simulink model "taetEMIL"  (R2021a)
settings: Solver=VariableStepAuto  StartTime=0.0  StopTime=2* 60*60  RelTol=1e-3
values from neighbouring files (symbols this model uses):
  Battery_Capacity = 100000    [load_global_variables.m]
  SOC_Start = 50    [load_global_variables.m]
  T_bat = 30*60    (= 1800)    [load_global_variables.m]
libraries: simulink x1
settings Model: Creator=cm  LastModifiedBy=cm

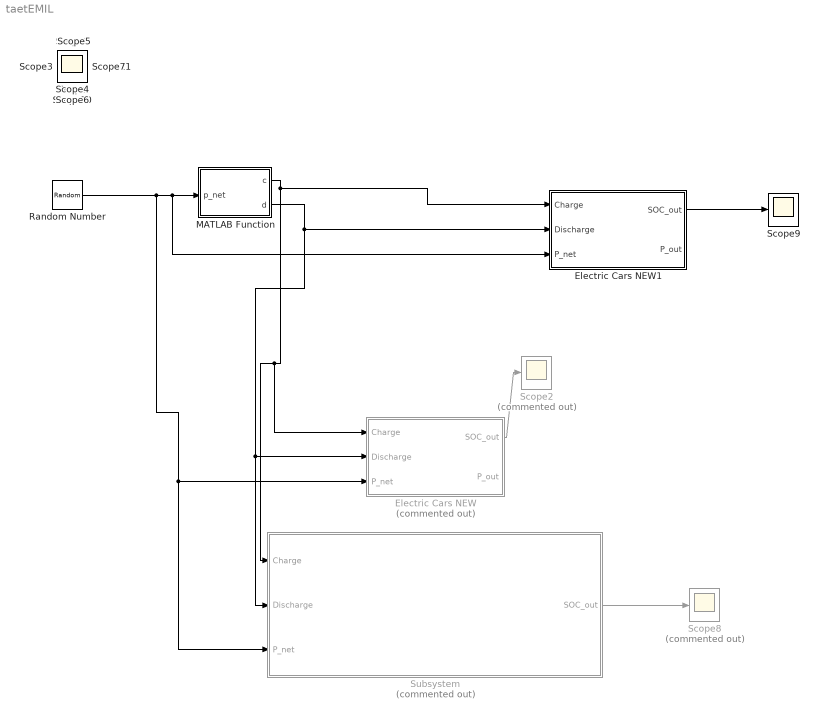
== system taetEMIL ==
  Electric Cars NEW : Subsystem  Commented=on
  Electric Cars NEW1 : Subsystem
  MATLAB Function : MATLAB Function  TreatAsAtomicUnit=on
  Random Number : RandomNumber  Variance=1000  SampleTime=10*60
  Scope2 : Scope  Commented=on
  Scope8 : Scope  Commented=on
  Scope{,1,3..7,9..11} (10 alike) : Scope
  Subsystem : Subsystem  Commented=on
  wires:
  MATLAB Function/1(c) -> Electric Cars NEW1/1(Charge), Subsystem/1(Charge), Electric Cars NEW/1(Charge)
  MATLAB Function/2(d) -> Electric Cars NEW1/2(Discharge), Subsystem/2(Discharge), Electric Cars NEW/2(Discharge)
  Electric Cars NEW/1(SOC_out) -> Scope2/1
  Random Number/1 -> Subsystem/3(P_net), Electric Cars NEW/3(P_net), Electric Cars NEW1/3(P_net), MATLAB Function/1(p_net)
  Subsystem/1(SOC_out) -> Scope8/1
  Electric Cars NEW1/1(SOC_out) -> Scope9/1

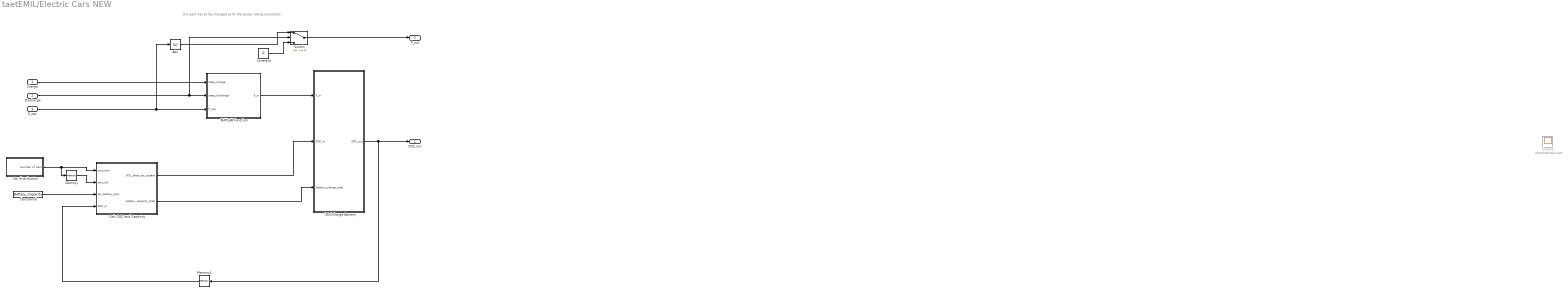
== system taetEMIL/Electric Cars NEW ==
  note: this part has to be changed to fit the power rating constraint
  Charge : Inport
  Discharge : Inport  Port=2
  P_net : Inport  Port=3
  (Dis)Charge Battery : Subsystem
  Abs : Abs
  Calc SOC and Capacity : MATLAB Function  TreatAsAtomicUnit=on
  Car distribution : Subsystem  TreatAsAtomicUnit=on
  Constant : Constant  Value=0
  Constant6 : Constant  Value=Battery_Capacity
  MATLAB Function : MATLAB Function  TreatAsAtomicUnit=on
  Memory : Memory  InitialCondition=100
  Memory1 : Memory  InitialCondition=SOC_Start
  Scope9 : Scope  Commented=on
  Switch : Switch  Criteria=u2 ~= 0
  SOC_out : Outport
  P_out : Outport  Port=2
  wires:
  Car distribution/1(Number of Cars) -> Memory/1, Calc SOC and Capacity/1(cars_new)
  Memory/1 -> Calc SOC and Capacity/2(cars_old)
  Constant6/1 -> Calc SOC and Capacity/3(car_battery_size)
  Memory1/1 -> Calc SOC and Capacity/4(SOC_in)
  MATLAB Function/1(P_in) -> (Dis)Charge Battery/1(P_in)
  Calc SOC and Capacity/1(SOC_after_car_update) -> (Dis)Charge Battery/2(SOC_in)
  Calc SOC and Capacity/2(battery_capacity_total) -> (Dis)Charge Battery/3(battery_charge_total)
  P_net/1 -> Abs/1, MATLAB Function/3(P_net)
  Discharge/1 -> Switch/2, MATLAB Function/2(state_discharge)
  Charge/1 -> MATLAB Function/1(state_charge)
  (Dis)Charge Battery/1(SOC_out) -> Memory1/1, SOC_out/1
  Abs/1 -> Switch/1
  Constant/1 -> Switch/3
  Switch/1 -> P_out/1

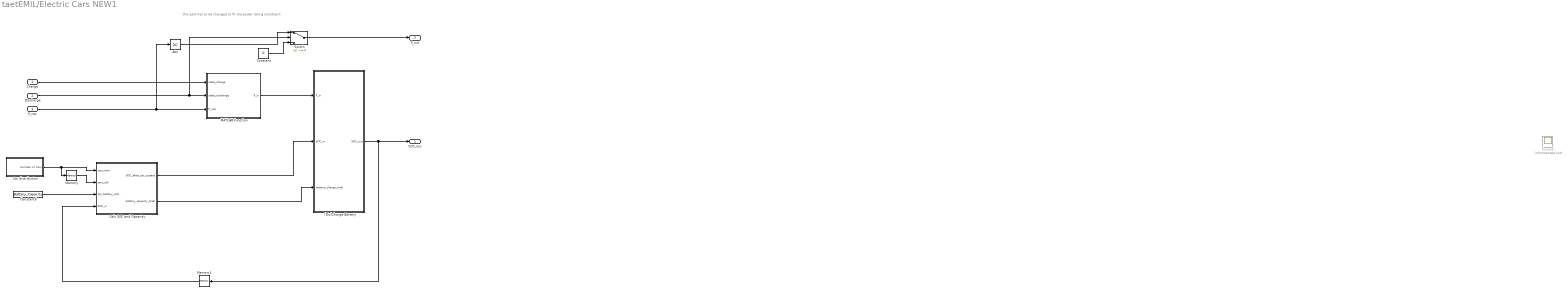
== system taetEMIL/Electric Cars NEW1 ==
  note: this part has to be changed to fit the power rating constraint
  Charge : Inport
  Discharge : Inport  Port=2
  P_net : Inport  Port=3
  (Dis)Charge Battery : Subsystem
  Abs : Abs
  Calc SOC and Capacity : MATLAB Function  TreatAsAtomicUnit=on
  Car distribution : Subsystem  TreatAsAtomicUnit=on
  Constant : Constant  Value=0
  Constant6 : Constant  Value=Battery_Capacity
  MATLAB Function : MATLAB Function  TreatAsAtomicUnit=on
  Memory : Memory  InitialCondition=1
  Memory1 : Memory  InitialCondition=SOC_Start
  Scope9 : Scope  Commented=on
  Switch : Switch  Criteria=u2 ~= 0
  SOC_out : Outport
  P_out : Outport  Port=2
  wires:
  Car distribution/1(Number of Cars) -> Memory/1, Calc SOC and Capacity/1(cars_new)
  Memory/1 -> Calc SOC and Capacity/2(cars_old)
  Constant6/1 -> Calc SOC and Capacity/3(car_battery_size)
  Memory1/1 -> Calc SOC and Capacity/4(SOC_in)
  MATLAB Function/1(P_in) -> (Dis)Charge Battery/1(P_in)
  Calc SOC and Capacity/1(SOC_after_car_update) -> (Dis)Charge Battery/2(SOC_in)
  Calc SOC and Capacity/2(battery_capacity_total) -> (Dis)Charge Battery/3(battery_charge_total)
  P_net/1 -> Abs/1, MATLAB Function/3(P_net)
  Discharge/1 -> Switch/2, MATLAB Function/2(state_discharge)
  Charge/1 -> MATLAB Function/1(state_charge)
  (Dis)Charge Battery/1(SOC_out) -> Memory1/1, SOC_out/1
  Abs/1 -> Switch/1
  Constant/1 -> Switch/3
  Switch/1 -> P_out/1

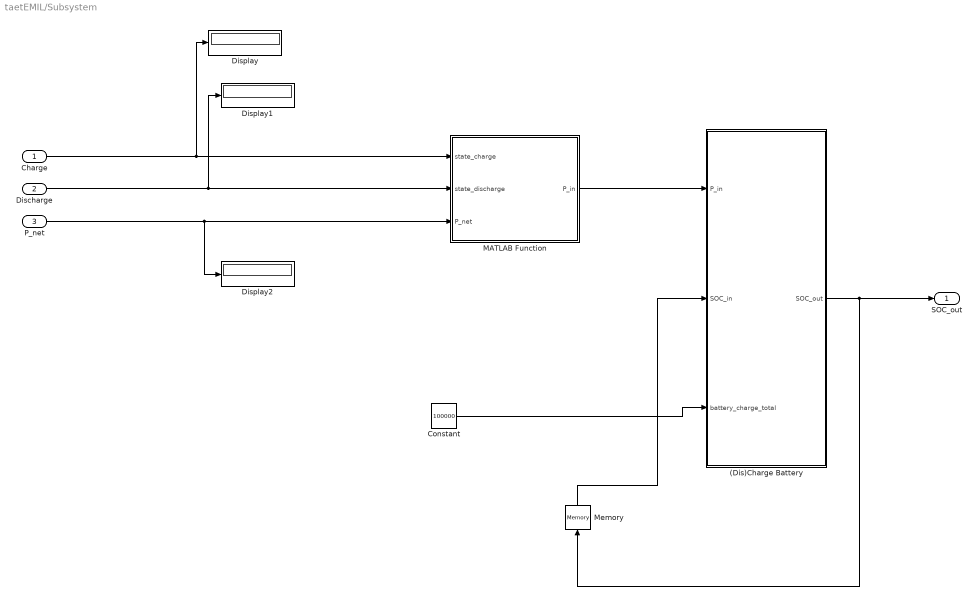
== system taetEMIL/Subsystem ==
  Charge : Inport
  Discharge : Inport  Port=2
  P_net : Inport  Port=3
  (Dis)Charge Battery : Subsystem
  Constant : Constant  Value=100000
  Display : Display
  Display1 : Display
  Display2 : Display
  MATLAB Function : MATLAB Function  TreatAsAtomicUnit=on
  Memory : Memory  InitialCondition=50
  SOC_out : Outport
  wires:
  Charge/1 -> Display/1, MATLAB Function/1(state_charge)
  MATLAB Function/1(P_in) -> (Dis)Charge Battery/1(P_in)
  P_net/1 -> Display2/1, MATLAB Function/3(P_net)
  Discharge/1 -> Display1/1, MATLAB Function/2(state_discharge)
  Memory/1 -> (Dis)Charge Battery/2(SOC_in)
  (Dis)Charge Battery/1(SOC_out) -> Memory/1, SOC_out/1
  Constant/1 -> (Dis)Charge Battery/3(battery_charge_total)

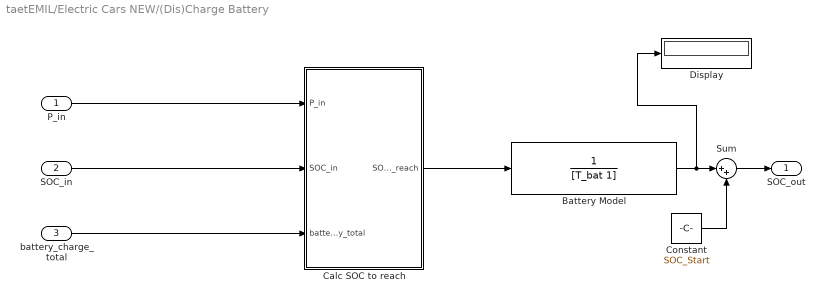
== system taetEMIL/Electric Cars NEW/(Dis)Charge Battery ==
  P_in : Inport
  SOC_in : Inport  Port=2
  battery_charge_total : Inport  Port=3
  Battery Model : TransferFcn  Numerator=1  Denominator=[T_bat 1]
  Calc SOC to reach : MATLAB Function  TreatAsAtomicUnit=on
  Constant : Constant  Value=SOC_Start
  Display : Display
  Sum : Sum  Inputs=|++
  SOC_out : Outport
  wires:
  Calc SOC to reach/1(SOC_to_reach) -> Battery Model/1
  P_in/1 -> Calc SOC to reach/1(P_in)
  SOC_in/1 -> Calc SOC to reach/2(SOC_in)
  battery_charge_total/1 -> Calc SOC to reach/3(battery_capacity_total)
  Sum/1 -> SOC_out/1
  Battery Model/1 -> Display/1, Sum/1
  Constant/1 -> Sum/2

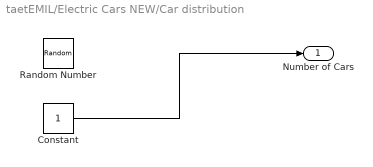
== system taetEMIL/Electric Cars NEW/Car distribution ==
  Constant : Constant
  Random Number : RandomNumber  Mean=50  Variance=15  SampleTime=10*60
  Number of Cars : Outport
  wires:
  Constant/1 -> Number of Cars/1

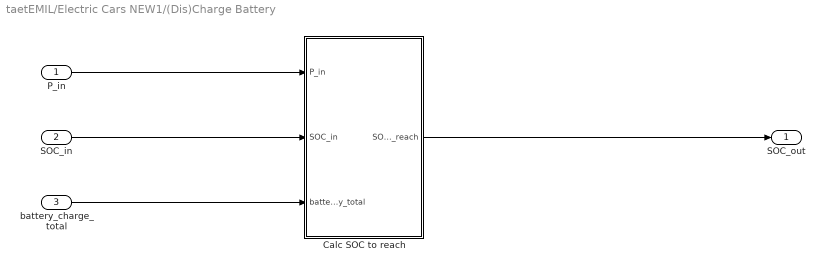
== system taetEMIL/Electric Cars NEW1/(Dis)Charge Battery ==
  P_in : Inport
  SOC_in : Inport  Port=2
  battery_charge_total : Inport  Port=3
  Calc SOC to reach : MATLAB Function  TreatAsAtomicUnit=on
  SOC_out : Outport
  wires:
  P_in/1 -> Calc SOC to reach/1(P_in)
  SOC_in/1 -> Calc SOC to reach/2(SOC_in)
  battery_charge_total/1 -> Calc SOC to reach/3(battery_capacity_total)
  Calc SOC to reach/1(SOC_to_reach) -> SOC_out/1

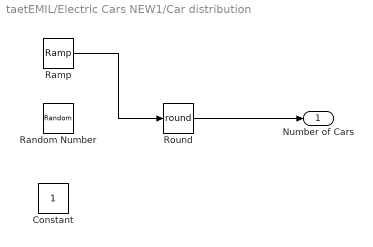
== system taetEMIL/Electric Cars NEW1/Car distribution ==
  Constant : Constant
  Ramp : simulink/Sources/Ramp  slope=0.01  start=1  InitialOutput=1
  Random Number : RandomNumber  Mean=1  Variance=2  SampleTime=60*15
  Round : Rounding  Operator=round
  Number of Cars : Outport
  wires:
  Round/1 -> Number of Cars/1
  Ramp/1 -> Round/1

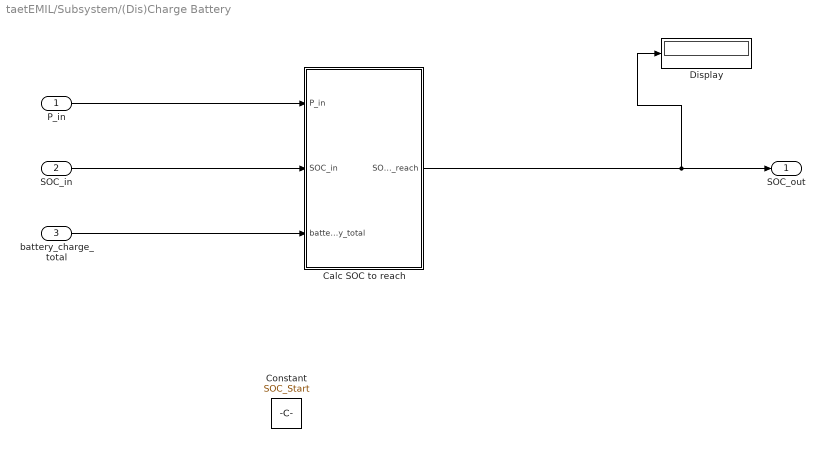
== system taetEMIL/Subsystem/(Dis)Charge Battery ==
  P_in : Inport
  SOC_in : Inport  Port=2
  battery_charge_total : Inport  Port=3
  Calc SOC to reach : MATLAB Function  TreatAsAtomicUnit=on
  Constant : Constant  Value=SOC_Start
  Display : Display
  SOC_out : Outport
  wires:
  battery_charge_total/1 -> Calc SOC to reach/3(battery_capacity_total)
  Calc SOC to reach/1(SOC_to_reach) -> SOC_out/1, Display/1
  SOC_in/1 -> Calc SOC to reach/2(SOC_in)
  P_in/1 -> Calc SOC to reach/1(P_in)

== matlab function taetEMIL/Subsystem/(Dis)Charge Battery/Calc SOC to reach ==
  data: P_in input; SOC_to_reach output; SOC_in input; battery_capacity_total input
function SOC_to_reach = fcn(P_in, SOC_in, battery_capacity_total)


charge_current = SOC_in/100*battery_capacity_total %[Wh]

charge_to_reach = P_in + charge_current

SOC_to_reach = charge_to_reach/battery_capacity_total  * 100


end

== matlab function taetEMIL/MATLAB Function ==
  data: p_net input; c output; d output
function [c,d] = fcn(p_net)
c= 0;
d = 0;

if p_net > 0 
    c = 1;
else
    d = 1;
end

== matlab function taetEMIL/Subsystem/MATLAB Function ==
  data: state_charge input; P_in output; state_discharge input; P_net input
function P_in = fcn(state_charge, state_discharge, P_net)

% function takes care that P_in is negative if we discharge and positive if
% we charge

if state_charge ~= 0
    P_in = abs(P_net);
elseif state_discharge ~= 0
    P_in = -abs(P_net);
else
    P_in = 0;
end

== matlab function taetEMIL/Electric Cars NEW1/(Dis)Charge Battery/Calc SOC to reach ==
  data: P_in input; SOC_to_reach output; SOC_in input; battery_capacity_total input
function SOC_to_reach = fcn(P_in, SOC_in, battery_capacity_total)

charge_current = SOC_in/100*battery_capacity_total; %[Wh]

charge_to_reach = P_in + charge_current;

SOC_to_reach = charge_to_reach/battery_capacity_total * 100;

== matlab function taetEMIL/Electric Cars NEW1/Calc SOC and Capacity ==
  data: cars_new input; SOC_after_car_update output; cars_old input; car_battery_size input; SOC_in input; battery_capacity_total output
function [SOC_after_car_update, battery_capacity_total]  = fcn(cars_new, cars_old, car_battery_size, SOC_in)

% For now we we see the cars as one and just a distribution over all
% IDEA:
    % We could work with cars as an array, each car is an element of the array
    % is a car. If the car is not in the charger the specific element in the
    % array is 0 otherwise it indicates the SOC.
    % Then we need a Controller in the Electric car model which loads the cars
    % individually

if cars_old == cars_new
    SOC_after_car_update = SOC_in;
elseif cars_old < cars_new
    % more cars
    % Calculate SOC of new cars randomly
    std_dev = 15;
    mean = 35;
    SOC_new = std_dev.*randn(1) + mean;
    
    if SOC_new <= 0
        % might happen because of normal distribution
        SOC_new = 1;
    end
    
    % Calculate new battery charge
    num_new_cars = cars_new - cars_old;
    capacity_new_cars = SOC_new/100 * car_battery_size * num_new_cars;
    
    capacity_old_cars = SOC_in/100 * car_battery_size * cars_old;
    
    % Calc SOC = (cap_new + cap_old) / total_cap * 100%
    SOC_after_car_update = (capacity_old_cars+capacity_new_cars)/(car_battery_size*cars_new) * 100;
    
elseif cars_old > cars_new
    % less cars
    SOC_after_car_update = SOC_in; % dont know how to do it otherwise, ideas welcome
    

else 
    % should not happen
    error('In Electric Cars/SOCcalc: unexpected case')
    SOC_after_car_update = SOC_in;
end

battery_capacity_total = car_battery_size * cars_new;

== matlab function taetEMIL/Electric Cars NEW1/MATLAB Function ==
  data: state_charge input; P_in output; state_discharge input; P_net input
function P_in = fcn(state_charge, state_discharge, P_net)

% function takes care that P_in is negative if we discharge and positive if
% we charge

if state_charge == 1
    P_in = abs(P_net);
elseif state_discharge == 1
    P_in = -abs(P_net);
else
    P_in = 0;
end

== matlab function taetEMIL/Electric Cars NEW/Calc SOC and Capacity ==
  data: cars_new input; SOC_after_car_update output; cars_old input; car_battery_size input; SOC_in input; battery_capacity_total output
function [SOC_after_car_update, battery_capacity_total]  = fcn(cars_new, cars_old, car_battery_size, SOC_in)

% For now we we see the cars as one and just a distribution over all
% IDEA:
    % We could work with cars as an array, each car is an element of the array
    % is a car. If the car is not in the charger the specific element in the
    % array is 0 otherwise it indicates the SOC.
    % Then we need a Controller in the Electric car model which loads the cars
    % individually

if cars_old == cars_new
    disp('same')
    SOC_after_car_update = SOC_in;
elseif cars_old < cars_new
    % more cars
    % Calculate SOC of new cars randomly
    disp('more')
    std_dev = 15;
    mean = 35;
    SOC_new = std_dev.*randn(1) + mean;
    
    if SOC_new <= 0
        % might happen because of normal distribution
        SOC_new = 1;
    end
    
    % Calculate new battery charge
    num_new_cars = cars_new - cars_old;
    capacity_new_cars = SOC_new/100 * car_battery_size * num_new_cars;
    
    capacity_old_cars = SOC_in/100 * car_battery_size * cars_old;
    
    % Calc SOC = (cap_new + cap_old) / total_cap * 100%
    SOC_after_car_update = (capacity_old_cars+capacity_new_cars)/(car_battery_size*cars_new) * 100
    
elseif cars_old > cars_new
    % less cars
    disp('less')
    SOC_after_car_update = SOC_in % dont know how to do it otherwise, ideas welcome
    

else 
    % should not happen
    error('In Electric Cars/SOCcalc: unexpected case')
    SOC_after_car_update = SOC_in;
end

battery_capacity_total = car_battery_size * cars_new;


SOC_after_car_update

if SOC_after_car_update > 100
    disp('error soc')
%     error('fuck')
elseif SOC_after_car_update <= 0.5
    disp('error soc')
%     error('fuck')
end

== matlab function taetEMIL/Electric Cars NEW/(Dis)Charge Battery/Calc SOC to reach ==
  data: P_in input; SOC_to_reach output; SOC_in input; battery_capacity_total input
function SOC_to_reach = fcn(P_in, SOC_in, battery_capacity_total)

charge_current = SOC_in/100*battery_capacity_total %[Wh]

charge_to_reach = P_in + charge_current

SOC_to_reach = charge_to_reach/battery_capacity_total  * 100

if SOC_to_reach > 100
%     error('SOC to big')
elseif SOC_to_reach < 10
    disp('too small')
end

== matlab function taetEMIL/Electric Cars NEW/MATLAB Function ==
  data: state_charge input; P_in output; state_discharge input; P_net input
function P_in = fcn(state_charge, state_discharge, P_net)

% function takes care that P_in is negative if we discharge and positive if
% we charge

if state_charge == 1
    P_in = abs(P_net);
elseif state_discharge == 1
    P_in = -abs(P_net);
else
    P_in = 0;
end
